simulink model "lab1_1_discrete"  (R2017b)
settings: Solver=ode45  StartTime=0.0  StopTime=10.0  RelTol=1e-3
undefined symbols (not defined in the file): DiscIntNeverNeededParam
settings Model: Creator=user  LastModifiedBy=HONOR
settings DataIOCC: LimitDataPoints=on  SaveFormat=Array
settings OptimizationCC: BlockReduction=off  BooleanDataType=off  LifeSpan=inf
settings DebuggingCC: SaveWithParameterizedLinksMsg=none  UnderspecifiedInitializationDetection=Classic  MergeDetectMultiDrivingBlocksExec=none  SignalResolutionControl=TryResolveAllWithWarning  SFUnexpectedBacktrackingDiag=warning  SFNoUnconditionalDefaultTransitionDiag=warning  SFExecutionAtInitializationDiag=none
settings HardwareCC: ProdBitPerPointer=32  ProdBitPerSizeT=32  ProdBitPerPtrDiffT=32  ProdLargestAtomicFloat=None  ProdIntDivRoundTo=Undefined  ProdEndianess=Unspecified  ProdWordSize=32  ProdHWDeviceType=32-bit Generic  TargetUnknown=on
settings ModelReferenceCC: PropagateSignalLabelsOutOfModel=off
settings CodeAppCC: StateflowObjectComments=on
settings GRTTargetCC: TargetLangStandard=C89/C90 (ANSI)  GeneratePreprocessorConditionals=Disable all
settings ConfigComp: CovMetricSettings=dw  CovHtmlReporting=on  CovSaveCumulativeToWorkspaceVar=on  CovSaveSingleToWorkspaceVar=on  CovExternalEMLEnable=off  CovSFcnEnable=off

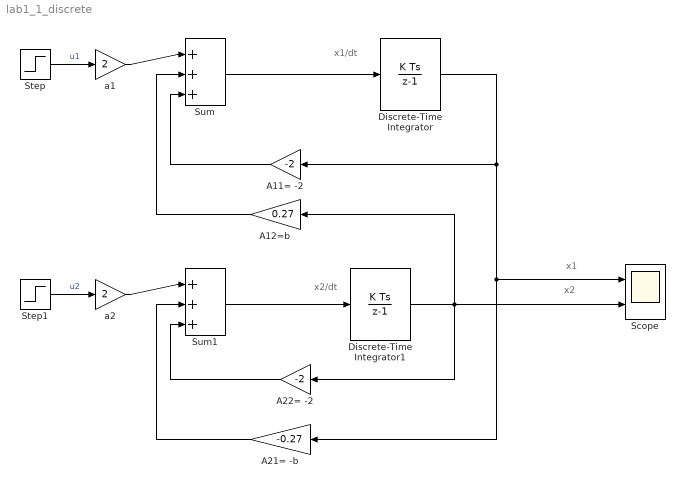
== system lab1_1_discrete ==
  note: x2
  note: x2/dt
  note: x1
  note: x1/dt
  A11= -2 : Gain  Gain=-2
  A12=b : Gain  Gain=0.27
  "A21= -b " : Gain  Gain=-0.27
  A22= -2 : Gain  Gain=-2
  Discrete-Time Integrator : DiscreteIntegrator  InitialConditionSetting=State (most efficient)  SampleTime=1.3  ICPrevOutput=DiscIntNeverNeededParam  ICPrevScaledInput=DiscIntNeverNeededParam
  Discrete-Time Integrator1 : DiscreteIntegrator  InitialConditionSetting=State (most efficient)  SampleTime=1.3  ICPrevOutput=DiscIntNeverNeededParam  ICPrevScaledInput=DiscIntNeverNeededParam
  Scope : Scope  NumInputPorts=2
  Step : Step  Time=0  After=0  SampleTime=0.15
  Step1 : Step  Time=0  SampleTime=0.15
  Sum : Sum  Inputs=|+++
  Sum1 : Sum  Inputs=|+++
  a1 : Gain  Gain=2
  a2 : Gain  Gain=2
  wires:
  Sum/1 -> Discrete-Time Integrator/1
  Sum1/1 -> Discrete-Time Integrator1/1
  Discrete-Time Integrator/1 -> Scope/1, "A21= -b "/1, A11= -2/1
  A11= -2/1 -> Sum/3
  Discrete-Time Integrator1/1 -> A12=b/1, Scope/2, A22= -2/1
  A12=b/1 -> Sum/2
  A22= -2/1 -> Sum1/3
  "A21= -b "/1 -> Sum1/2
  Step/1 -> a1/1  "u1"
  Step1/1 -> a2/1  "u2"
  a2/1 -> Sum1/1
  a1/1 -> Sum/1
